simulink model "robustTrackingModel"  (R2019b)
settings: Solver=VariableStepAuto  StartTime=0.0  StopTime=10  RelTol=1e-3
values from neighbouring files (symbols this model uses):
  encGain = (2*pi)/4096    (= 0.00153398078789)    [DC_Motor_Analysis.m]    (also in Part2.m; Part3.m; lqrPoles.mat; robust.mat)
  K = K_tilde(1:2)    [DC_Motor_Analysis.m]    (also in Part3.m = double(linsolve(meatMat, potatoesMat)))
  Ka = K_tilde(end)    [DC_Motor_Analysis.m]
  stepInput = 0    [DC_Motor_Analysis.m]
settings Model: Creator=justinf  LastModifiedBy=justinf

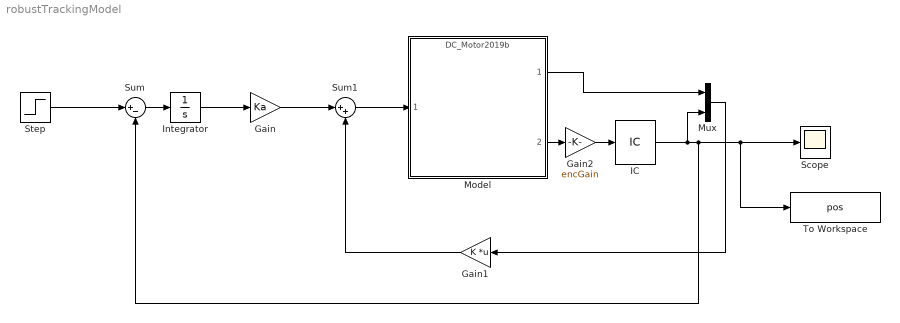
== system robustTrackingModel ==
  Gain : Gain  Gain=Ka
  Gain1 : Gain  Gain=K  Multiplication=Matrix(K*u)
  Gain2 : Gain  Gain=encGain
  IC : InitialCondition  Value=-1
  Integrator : Integrator
  Model : ModelReference  ModelNameDialog=DC_Motor2019b.slxp  ModelReferenceVersion=1.20  CopyOfModelProtected=on
  Mux : Mux  Inputs=2
  Scope : Scope
  Step : Step  Time=0  After=stepInput  SampleTime=0
  Sum : Sum  Inputs=|+-
  Sum1 : Sum  Inputs=|++
  To Workspace : ToWorkspace  VariableName=pos  SampleTime=-1
  wires:
  Model/1 -> Mux/1
  Model/2 -> Gain2/1
  Mux/1 -> Gain1/1
  Integrator/1 -> Gain/1
  Gain/1 -> Sum1/1
  Sum1/1 -> Model/1
  Gain1/1 -> Sum1/2
  Sum/1 -> Integrator/1
  Step/1 -> Sum/1
  Gain2/1 -> IC/1
  IC/1 -> To Workspace/1, Scope/1, Sum/2, Mux/2
